simulink model "model_2_4"  (R2021b)
settings: Solver=FixedStepAuto  StartTime=0.0  StopTime=10  FixedStep=0.0005  RelTol=1e-3
settings Model: Creator=den  LastModifiedBy=den

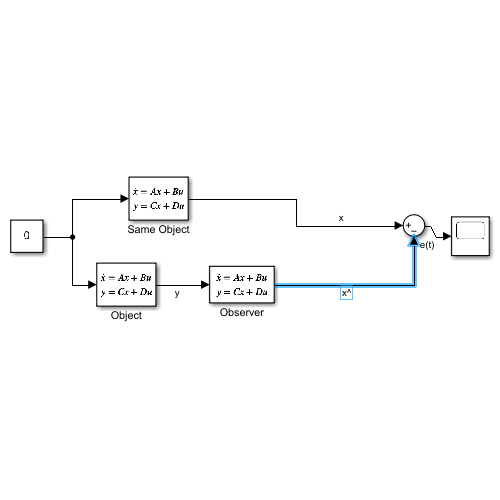
[thumbnail: Simulink's stored preview of the top-level diagram]
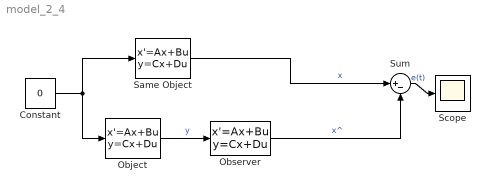
== system model_2_4 ==
  Constant : Constant  Value=0
  Object : StateSpace  A=[0 5 0 0; -5 0 0 0; 0 0 0 1; 0 0 -1 0]  B=[0; 0; 0; 0]  C=[0 9 1 0]  D=0  InitialCondition=[1;1;1;1]
  Observer : StateSpace  A=[0 269/12 209/108 0; -5 -7/6 -7/54 0; 0 -303/2 -101/6 1; 0 -573/4 -203/12 0]  B=[-209/108 ;7/54 ;101/6; 191/12]  C=[1 0 0 0; 0 1 0 0; 0 0 1 0; 0 0 0 1]  D=[0;0;0;0]  InitialCondition=[2;0;0;-1]
  Same Object : StateSpace  A=[0 5 0 0; -5 0 0 0; 0 0 0 1; 0 0 -1 0]  B=[0; 0; 0; 0]  C=[1 0 0 0; 0 1 0 0; 0 0 1 0; 0 0 0 1]  D=[0;0;0;0]  InitialCondition=[1;1;1;1]
  Scope : Scope
  Sum : Sum  Inputs=|+-
  wires:
  Object/1 -> Observer/1  "y"
  Observer/1 -> Sum/2  "x^"
  Constant/1 -> Same Object/1, Object/1
  Same Object/1 -> Sum/1  "x"
  Sum/1 -> Scope/1  "e(t)"
